simulink library "asbCubeSatDynamicsLib"  (R2019a)
settings: Solver=VariableStepAuto  StartTime=0.0  StopTime=10.0  RelTol=1e-3
undefined symbols (not defined in the file): Earth, initCond, WGS84
libraries: aerolib6dof2 x1, asbCubeSatBlockLib x1, sharedtransform x1
settings Model: Creator=The MathWorks, Inc.  LastModifiedBy=The MathWorks, Inc.
settings DataIOCC: ReturnWorkspaceOutputs=off
settings DebuggingCC: ArithmeticOperatorsInVariantConditions=warning

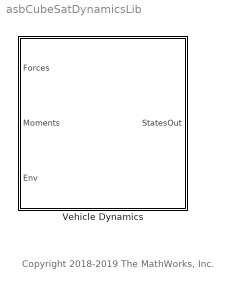
== system asbCubeSatDynamicsLib ==
  note: Copyright 2018-2019 The MathWorks, Inc.
  Vehicle Dynamics : Subsystem

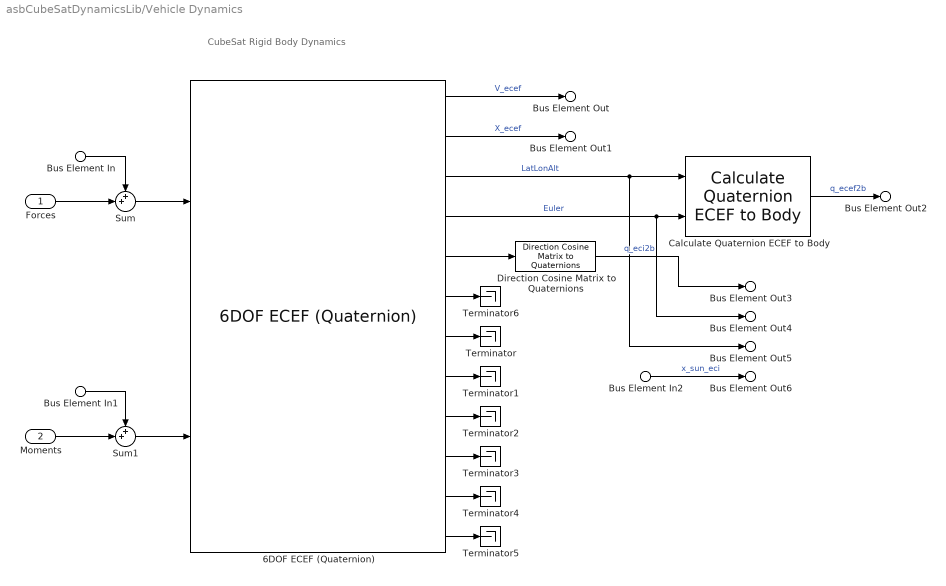
== system asbCubeSatDynamicsLib/Vehicle Dynamics ==
  note: CubeSat Rigid Body Dynamics
  Forces : Inport  RequirementInfo={} %GIDa_3bff085b_b60a_4e83_9a79_ee4d75de2c18
  Moments : Inport  RequirementInfo={} %GIDa_de23e7b3_b020_4a27_8ea7_dbdbe2a400f3  Port=2
  Bus Element In : Inport  Port=3  PortName=Env  Element=envForces_body
  Bus Element In1 : Inport  Port=3  PortName=Env  Element=envTorques_body
  Bus Element In2 : Inport  Port=3  PortName=Env  Element=x_sun_eci
  6DOF ECEF (Quaternion) : aerolib6dof2/6DOF ECEF (Quaternion)  units=Metric (MKS)  mtype=Fixed  xg_0=initCond.lla  Vm_0=initCond.uvw  eul_0=initCond.euler*pi/180  pm_0=initCond.pqr*pi/180  mass_0=vehicle.mass  mass_e=0.5  mass_f=2.0  inertia=vehicle.inertia  inertia_e=eye(3)  inertia_f=2*eye(3)  vre_flag=on  abi_flag=off  ptype=Earth (WGS84)  R=6378137  F=1/298.257223563  w_E=7292115e-11  angle_in=Internal  LG0=initCond.EarthProps.LG  quat_statename=''  pm_statename=''  Vm_statename=''  posECEF_statename=''  posECI_statename=''  LG_statename=''  mass_statename=''
      settings: SourceProductName=Aerospace Blockset  SourceProductBaseCode=AE
  Calculate Quaternion ECEF to Body : asbCubeSatBlockLib/Axes Transformations/Coordinate System Transformations/Calculate Quaternion ECEF to Body  SystemSampleTime=-1
  Direction Cosine Matrix to Quaternions : sharedtransform/Direction Cosine Matrix  to Quaternions  RequirementInfo={} %GIDa_f6acb073_5fc2_4121_8cd8_59723b754a8d  aMode=aMode  action=None  tolerance=eps(2)
      settings: SourceProductName=Aerospace Blockset  SourceProductBaseCode=AE
  Sum : Sum  RequirementInfo={} %GIDa_93ce11cd_3bb8_4d3a_a1de_f1041c0e8540  Inputs=++|
  Sum1 : Sum  RequirementInfo={} %GIDa_6da28457_7485_4e17_8924_3ed2b0e1d29f  Inputs=++|
  Terminator{,1..6} (7 alike) : Terminator
      Terminator settings: RequirementInfo={} %GIDa_956375aa_2a0c_4f1b_aae6_0780c334247b
      Terminator1 settings: RequirementInfo={} %GIDa_f1298799_1a13_4857_a66c_aafd0a82e29e
      Terminator2 settings: RequirementInfo={} %GIDa_2b2e7357_3abf_4963_8534_2f632ac88ef5
      Terminator3 settings: RequirementInfo={} %GIDa_df46343b_422d_459d_94ff_228587090c47
      Terminator4 settings: RequirementInfo={} %GIDa_76e8a3d8_914f_4b26_982c_b95e0f910c39
      Terminator5 settings: RequirementInfo={} %GIDa_e819ad6a_8486_4847_824c_1dc065b780ef
      Terminator6 settings: RequirementInfo={} %GIDa_d53ded5e_1d3b_4065_a418_ae6886d8bb0a
  Bus Element Out : Outport  PortName=StatesOut  Element=V_ecef
  Bus Element Out1 : Outport  PortName=StatesOut  Element=X_ecef
  Bus Element Out2 : Outport  PortName=StatesOut  Element=q_ecef2b
  Bus Element Out3 : Outport  PortName=StatesOut  Element=q_eci2b
  Bus Element Out4 : Outport  PortName=StatesOut  Element=Euler
  Bus Element Out5 : Outport  PortName=StatesOut  Element=LatLonAlt
  Bus Element Out6 : Outport  PortName=StatesOut  Element=x_sun_eci
  wires:
  Sum1/1 -> 6DOF ECEF (Quaternion)/2
  Sum/1 -> 6DOF ECEF (Quaternion)/1
  6DOF ECEF (Quaternion)/3 -> Calculate Quaternion ECEF to Body/1, Bus Element Out5/1  "LatLonAlt"
  6DOF ECEF (Quaternion)/1 -> Bus Element Out/1  "V_ecef"
  Calculate Quaternion ECEF to Body/1 -> Bus Element Out2/1  "q_ecef2b"
  6DOF ECEF (Quaternion)/4 -> Calculate Quaternion ECEF to Body/2, Bus Element Out4/1  "Euler"
  Direction Cosine Matrix to Quaternions/1 -> Bus Element Out3/1  "q_eci2b"
  6DOF ECEF (Quaternion)/8 -> Terminator1/1
  6DOF ECEF (Quaternion)/6 -> Terminator6/1
  6DOF ECEF (Quaternion)/12 -> Terminator5/1
  6DOF ECEF (Quaternion)/7 -> Terminator/1
  6DOF ECEF (Quaternion)/11 -> Terminator4/1
  6DOF ECEF (Quaternion)/5 -> Direction Cosine Matrix to Quaternions/1
  6DOF ECEF (Quaternion)/9 -> Terminator2/1
  6DOF ECEF (Quaternion)/10 -> Terminator3/1
  6DOF ECEF (Quaternion)/2 -> Bus Element Out1/1  "X_ecef"
  Forces/1 -> Sum/2
  Bus Element In/1 -> Sum/1
  Bus Element In2/1 -> Bus Element Out6/1  "x_sun_eci"
  Bus Element In1/1 -> Sum1/1
  Moments/1 -> Sum1/2
